simulink model "celab1"  (R2023b)
settings: Solver=VariableStepAuto  StartTime=0.0  StopTime=120  RelTol=1e-3
settings Model: Creator=Lenovo  LastModifiedBy=Lenovo

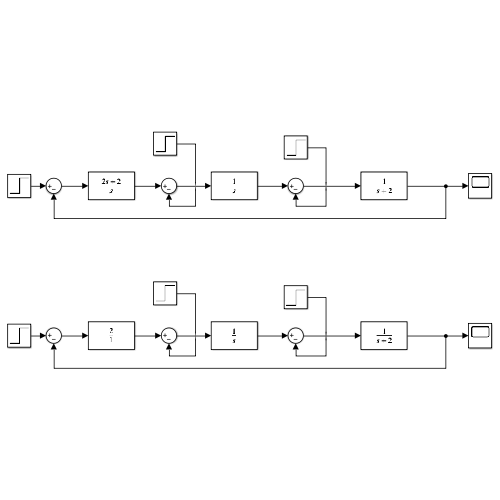
[thumbnail: Simulink's stored preview of the top-level diagram]
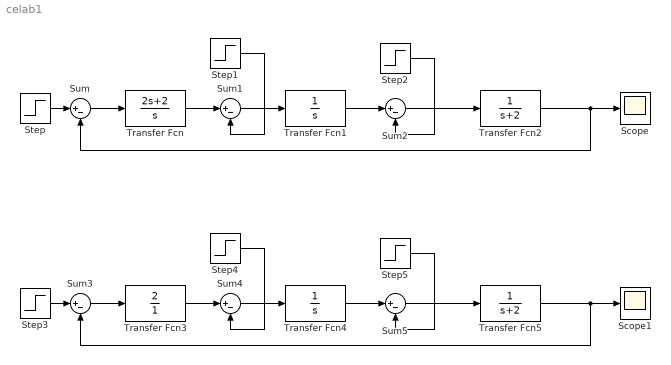
== system celab1 ==
  Scope : Scope
  Scope1 : Scope
  Step : Step  SampleTime=0
  Step1 : Step  Time=15  SampleTime=0
  Step2 : Step  Time=25  SampleTime=0
  Step3 : Step  SampleTime=0
  Step4 : Step  Time=15  SampleTime=0
  Step5 : Step  Time=25  SampleTime=0
  Sum{,1..5} (6 alike) : Sum  Inputs=|+-
  Transfer Fcn : TransferFcn  Numerator=[2 2]  Denominator=[1 0 ]
  Transfer Fcn1 : TransferFcn  Denominator=[1 0]
  Transfer Fcn2 : TransferFcn  Denominator=[1 2]
  Transfer Fcn3 : TransferFcn  Numerator=2  Denominator=1
  Transfer Fcn4 : TransferFcn  Denominator=[1 0]
  Transfer Fcn5 : TransferFcn  Denominator=[1 2]
  wires:
  Sum/1 -> Transfer Fcn/1
  Transfer Fcn/1 -> Sum1/1
  Sum1/1 -> Transfer Fcn1/1
  Transfer Fcn1/1 -> Sum2/1
  Sum2/1 -> Transfer Fcn2/1
  Transfer Fcn2/1 -> Sum/2, Scope/1
  Step/1 -> Sum/1
  Step1/1 -> Sum1/2
  Step2/1 -> Sum2/2
  Step4/1 -> Sum4/2
  Step5/1 -> Sum5/2
  Sum5/1 -> Transfer Fcn5/1
  Transfer Fcn3/1 -> Sum4/1
  Step3/1 -> Sum3/1
  Sum3/1 -> Transfer Fcn3/1
  Transfer Fcn5/1 -> Sum3/2, Scope1/1
  Sum4/1 -> Transfer Fcn4/1
  Transfer Fcn4/1 -> Sum5/1
